simulink model "ModDelta"  (R2015a)
settings: Solver=ode45  StartTime=0.0  StopTime=0.125  RelTol=1e-3
libraries: dsparch4 x1, dspsigops x1
settings Model: Creator=user  LastModifiedBy=user

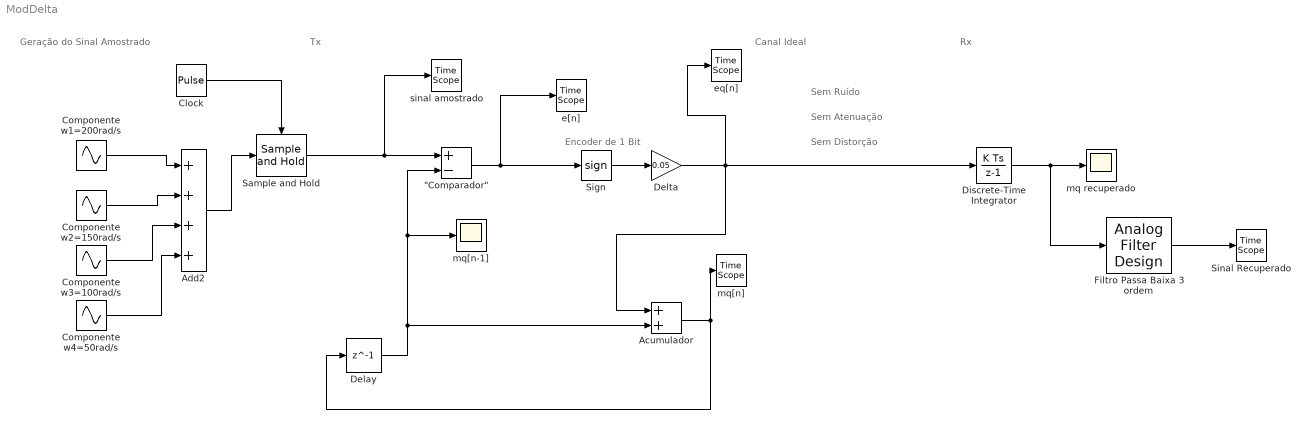
== system ModDelta ==
  note: Sem Ruído
  note: Encoder de 1 Bit
  note: Geração do Sinal Amostrado
  note: Tx
  note: Rx
  note: Canal Ideal
  note: Sem Atenuação
  note: Sem Distorção
  "\"Comparador\"" : Sum  Inputs=+-
  Acumulador : Sum
  Add2 : Sum  Inputs=++++
  Clock : DiscretePulseGenerator  PulseType=Time based  Period=0.0001  PulseWidth=5
  Componente w1=200rad/s : Sin  Amplitude=0.25  Frequency=200  SampleTime=0
  Componente w2=150rad/s : Sin  Amplitude=0.25  Frequency=150  SampleTime=0
  Componente w3=100rad/s : Sin  Amplitude=0.25  Frequency=100  SampleTime=0
  Componente w4=50rad/s : Sin  Amplitude=0.25  Frequency=50  SampleTime=0
  Delay : Delay  DelayLength=1  SampleTime=0.0001
  Delta : Gain  Gain=0.05
  Discrete-Time Integrator : DiscreteIntegrator  gainval=1/0.0001  InitialConditionSetting=State (most efficient)  SampleTime=0.0001
  Filtro Passa Baixa 3 ordem : dsparch4/Analog Filter Design  method=Butterworth  filttype=Lowpass  N=3  Wlo=250  Whi=80  Rp=2  Rs=40
  Sample and Hold : dspsigops/Sample and Hold  trig=Rising edge  initCond=0  latchinput=off
  Sign : Signum
  Sinal Recuperado : TimeScope
  e[n] : TimeScope
  eq[n] : TimeScope
  mq recuperado : Scope
      settings: TimeRange=0.1  YMin=-9.999999999999999e-05  YMax=0.0001  SaveName=ScopeData5
  mq[n-1] : Scope
      settings: SaveName=ScopeData3
  mq[n] : TimeScope
  sinal amostrado : TimeScope
  wires:
  "\"Comparador\""/1 -> Sign/1, e[n]/1
  Sign/1 -> Delta/1
  Acumulador/1 -> Delay/1, mq[n]/1
  Delay/1 -> Acumulador/2, "\"Comparador\""/2, mq[n-1]/1
  Clock/1 -> Sample and Hold/Trigger
  Delta/1 -> Acumulador/1, Discrete-Time Integrator/1, eq[n]/1
  Discrete-Time Integrator/1 -> Filtro Passa Baixa 3 ordem/1, mq recuperado/1
  Filtro Passa Baixa 3 ordem/1 -> Sinal Recuperado/1
  Componente w1=200rad/s/1 -> Add2/1
  Add2/1 -> Sample and Hold/1
  Componente w2=150rad/s/1 -> Add2/2
  Componente w3=100rad/s/1 -> Add2/3
  Componente w4=50rad/s/1 -> Add2/4
  Sample and Hold/1 -> "\"Comparador\""/1, sinal amostrado/1
